simulink model "FIR_FILTER_CASCADEFORM_7"  (R2020b)
settings: Solver=VariableStepAuto  StartTime=0.0  StopTime=10.0  RelTol=1e-3
settings Model: Creator=intel  LastModifiedBy=intel

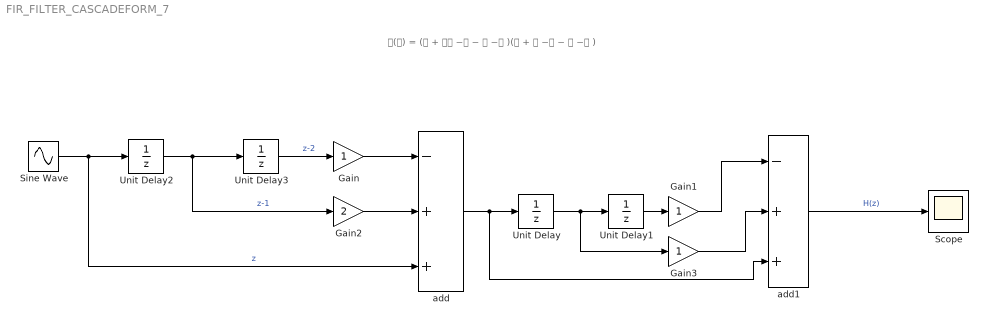
== system FIR_FILTER_CASCADEFORM_7 ==
  note: 𝐇(𝐳) = (𝟏 + 𝟐𝐳 −𝟏 − 𝐳 −𝟐 )(𝟏 + 𝐳 −𝟏 − 𝐳 −𝟐 )
  Gain : Gain
  Gain1 : Gain
  Gain2 : Gain  Gain=2
  Gain3 : Gain
  Scope : Scope
  Sine Wave : Sin  SampleTime=0
  Unit Delay{,1..3} (4 alike) : UnitDelay  SampleTime=-1  HasFrameUpgradeWarning=on
  add : Sum  Inputs=-++
  add1 : Sum  Inputs=-++
  wires:
  Sine Wave/1 -> Unit Delay2/1, add/3  "z"
  Gain2/1 -> add/2
  Gain/1 -> add/1
  Unit Delay2/1 -> Unit Delay3/1, Gain2/1  "z-1"
  Unit Delay3/1 -> Gain/1  "z-2"
  Unit Delay/1 -> Gain3/1, Unit Delay1/1
  add/1 -> add1/3, Unit Delay/1
  Unit Delay1/1 -> Gain1/1
  Gain1/1 -> add1/1
  add1/1 -> Scope/1  "H(z)"
  Gain3/1 -> add1/2
